simulink model "MSRE_final"  (R2017a)
settings: Solver=ode45  StartTime=0.0  StopTime=1500
values from neighbouring files (symbols this model uses):
  a_f = -11.034E-5    (= -0.00011034)    [Parameters_MSRE_cold_slug_U233.m]    (also in Parameters_MSRE_cold_slug_U235.m = -8.71e-05; Parameters_MSRE_pump_trip.m = -8.46e-05)
  a_g = -5.814E-5    (= -5.814e-05)    [Parameters_MSRE_cold_slug_U233.m]    (also in Parameters_MSRE_cold_slug_U235.m = -6.66e-05; Parameters_MSRE_pump_trip.m = -4.68e-05)
  beta = [0.00023,0.00079,0.00067,0.00073,0.00013,0.00009]    [Parameters_MSRE_cold_slug_U233.m]    (also in Parameters_MSRE_cold_slug_U235.m = [0.000223,0.001457,0.001307,0.002628,0.000766,0.00023]; Parameters_MSRE_pump_trip.m = [0.000215,0.00142,0.00127,0.00257,0.00075,0.00027])
  beta_t = sum(beta)    [Parameters_MSRE_cold_slug_U233.m]    (also in Parameters_MSRE_cold_slug_U235.m; Parameters_MSRE_pump_trip.m)
  hA_fg = 0.02*9/5    (= 0.036)    [Parameters_MSRE_cold_slug_U233.m]    (also in Parameters_MSRE_cold_slug_U235.m; Parameters_MSRE_pump_trip.m)
  hA_pn = ha_p/nn_s    (= 0.162)    [Parameters_MSRE_cold_slug_U233.m]    (also in Parameters_MSRE_cold_slug_U235.m; Parameters_MSRE_pump_trip.m)
  hA_rpn = h_roverall*A_rad/nn_rs    (= 0.0170417629704)    [Parameters_MSRE_cold_slug_U233.m]    (also in Parameters_MSRE_cold_slug_U235.m; Parameters_MSRE_pump_trip.m = 0.0166958844645)
  hA_rsn = h_roverall*A_rad/nn_rs    (= 0.0170417629704)    [Parameters_MSRE_cold_slug_U233.m]    (also in Parameters_MSRE_cold_slug_U235.m; Parameters_MSRE_pump_trip.m = 0.0166958844645)
  hA_sn = ha_s/nn_s    (= 0.0765)    [Parameters_MSRE_cold_slug_U233.m]    (also in Parameters_MSRE_cold_slug_U235.m; Parameters_MSRE_pump_trip.m)
  k_1 = 0.5    [Parameters_MSRE_cold_slug_U233.m]    (also in Parameters_MSRE_cold_slug_U235.m; Parameters_MSRE_pump_trip.m)
  k_2 = 0.5    [Parameters_MSRE_cold_slug_U233.m]    (also in Parameters_MSRE_cold_slug_U235.m; Parameters_MSRE_pump_trip.m)
  k_f1 = k_f/nn_f    (= 0.465)    [Parameters_MSRE_cold_slug_U233.m]    (also in Parameters_MSRE_cold_slug_U235.m; Parameters_MSRE_pump_trip.m)
  k_f2 = k_f/nn_f    (= 0.465)    [Parameters_MSRE_cold_slug_U233.m]    (also in Parameters_MSRE_cold_slug_U235.m; Parameters_MSRE_pump_trip.m)
  k_g = 0.07    [Parameters_MSRE_cold_slug_U233.m]    (also in Parameters_MSRE_cold_slug_U235.m; Parameters_MSRE_pump_trip.m)
  Lam = 4.0E-04    (= 0.0004)    [Parameters_MSRE_cold_slug_U233.m]    (also in Parameters_MSRE_cold_slug_U235.m = 0.00024; Parameters_MSRE_pump_trip.m = 0.00024)
  lam = [1.260E-02, 3.370E-02, 1.390E-01, 3.250E-01, 1.130E+00, 2.500E+00]    [Parameters_MSRE_cold_slug_U233.m]    (also in Parameters_MSRE_cold_slug_U235.m = [1.240E-02, 3.05E-02, 1.11E-01, 3.01E-01, 1.140E+00, 3.014E+; Parameters_MSRE_pump_trip.m)
  mcp_f1 = mn_f*scp_f    (= 1.52295504008)    [Parameters_MSRE_cold_slug_U233.m]    (also in Parameters_MSRE_cold_slug_U235.m; Parameters_MSRE_pump_trip.m = 1.32669270969)
  mcp_f2 = mn_f*scp_f    (= 1.52295504008)    [Parameters_MSRE_cold_slug_U233.m]    (also in Parameters_MSRE_cold_slug_U235.m; Parameters_MSRE_pump_trip.m = 1.32669270969)
  mcp_g1 = m_g*scp_g    (= 6.48)    [Parameters_MSRE_cold_slug_U233.m]    (also in Parameters_MSRE_cold_slug_U235.m; Parameters_MSRE_pump_trip.m)
  mcp_pn = mn_p*cp_p    (= 0.171274079686)    [Parameters_MSRE_cold_slug_U233.m]    (also in Parameters_MSRE_cold_slug_U235.m; Parameters_MSRE_pump_trip.m = 0.168097428848)
  mcp_rpn = mn_rp*cp_rp    (= 0.870039765806)    [Parameters_MSRE_cold_slug_U233.m]    (also in Parameters_MSRE_cold_slug_U235.m; Parameters_MSRE_pump_trip.m = 0.937931908109)
  mcp_rsn = mn_rs*scp_rs    (= 0.00358005261349)    [Parameters_MSRE_cold_slug_U233.m]    (also in Parameters_MSRE_cold_slug_U235.m; Parameters_MSRE_pump_trip.m)
  mcp_sn = mn_s*scp_s    (= 0.055247682268)    [Parameters_MSRE_cold_slug_U233.m]    (also in Parameters_MSRE_cold_slug_U235.m; Parameters_MSRE_pump_trip.m = 0.0595588455663)
  mcp_tn = m_tn*scp_t    (= 0.058453833323)    [Parameters_MSRE_cold_slug_U233.m]    (also in Parameters_MSRE_cold_slug_U235.m; Parameters_MSRE_pump_trip.m)
  mn_f = m_f/nn_f    (= 774.44955)    [Parameters_MSRE_cold_slug_U233.m]    (also in Parameters_MSRE_cold_slug_U235.m; Parameters_MSRE_pump_trip.m = 687.40554906)
  mn_p = m_p/nn_p    (= 87.0958961026)    [Parameters_MSRE_cold_slug_U233.m]    (also in Parameters_MSRE_cold_slug_U235.m; Parameters_MSRE_pump_trip.m = 87.0971133928)
  mn_rp = m_rp/nn_rp    (= 392.440128916)    [Parameters_MSRE_cold_slug_U233.m]    (also in Parameters_MSRE_cold_slug_U235.m; Parameters_MSRE_pump_trip.m)
  mn_rs = m_rs/nn_rs    (= 3.549878645)    [Parameters_MSRE_cold_slug_U233.m]    (also in Parameters_MSRE_cold_slug_U235.m; Parameters_MSRE_pump_trip.m)
  mn_s = m_s/nn_s    (= 24.9200190654)    [Parameters_MSRE_cold_slug_U233.m]    (also in Parameters_MSRE_cold_slug_U235.m; Parameters_MSRE_pump_trip.m)
  n_frac0 = 1    [Parameters_MSRE_cold_slug_U233.m]    (also in Parameters_MSRE_cold_slug_U235.m; Parameters_MSRE_pump_trip.m)
  P = 8    [Parameters_MSRE_cold_slug_U233.m]    (also in Parameters_MSRE_cold_slug_U235.m; Parameters_MSRE_pump_trip.m)
  T0_f1 = Tf_in + (T0_f2-Tf_in)/2    (= 643.33)    [Parameters_MSRE_cold_slug_U233.m]    (also in Parameters_MSRE_cold_slug_U235.m; Parameters_MSRE_pump_trip.m = 648.9)
  T0_f2 = 6.5444E+02    (= 654.44)    [Parameters_MSRE_cold_slug_U233.m]    (also in Parameters_MSRE_cold_slug_U235.m; Parameters_MSRE_pump_trip.m = 662.8)
  T0_g1 = T0_f1+(k_g*P/hA_fg)    (= 658.885555556)    [Parameters_MSRE_cold_slug_U233.m]    (also in Parameters_MSRE_cold_slug_U235.m; Parameters_MSRE_pump_trip.m = 664.455555556)
  T0_p1 = Tp_in - (Tp_in-T0_p4)/4    (= 648.885)    [Parameters_MSRE_cold_slug_U233.m]    (also in Parameters_MSRE_cold_slug_U235.m; Parameters_MSRE_pump_trip.m = 655.85)
  T0_p2 = Tp_in - 2*(Tp_in-T0_p4)/4    (= 643.33)    [Parameters_MSRE_cold_slug_U233.m]    (also in Parameters_MSRE_cold_slug_U235.m; Parameters_MSRE_pump_trip.m = 648.9)
  T0_p3 = Tp_in - 3*(Tp_in-T0_p4)/4    (= 637.775)    [Parameters_MSRE_cold_slug_U233.m]    (also in Parameters_MSRE_cold_slug_U235.m; Parameters_MSRE_pump_trip.m = 641.95)
  T0_p4 = Tf_in    (= 632.22)    [Parameters_MSRE_cold_slug_U233.m]    (also in Parameters_MSRE_cold_slug_U235.m; Parameters_MSRE_pump_trip.m = 635)
  T0_rp = Ts_in    (= 546.11)    [Parameters_MSRE_cold_slug_U233.m]    (also in Parameters_MSRE_cold_slug_U235.m; Parameters_MSRE_pump_trip.m = 551.7)
  T0_rs = 148.9    [Parameters_MSRE_cold_slug_U233.m]    (also in Parameters_MSRE_cold_slug_U235.m; Parameters_MSRE_pump_trip.m)
  T0_s1 = Ts_in + (T0_s4-Ts_in)/nn_s    (= 554.4425)    [Parameters_MSRE_cold_slug_U233.m]    (also in Parameters_MSRE_cold_slug_U235.m; Parameters_MSRE_pump_trip.m = 562.1)
  T0_s2 = Ts_in + 2*(T0_s4-Ts_in)/nn_s    (= 562.775)    [Parameters_MSRE_cold_slug_U233.m]    (also in Parameters_MSRE_cold_slug_U235.m; Parameters_MSRE_pump_trip.m = 572.5)
  T0_s3 = Ts_in + 3*(T0_s4-Ts_in)/nn_s    (= 571.1075)    [Parameters_MSRE_cold_slug_U233.m]    (also in Parameters_MSRE_cold_slug_U235.m; Parameters_MSRE_pump_trip.m = 582.9)
  T0_s4 = 5.7944E+02    (= 579.44)    [Parameters_MSRE_cold_slug_U233.m]    (also in Parameters_MSRE_cold_slug_U235.m; Parameters_MSRE_pump_trip.m = 593.3)
  T0_t1 = (T0_p1*hA_pn+T0_s3*hA_sn)/(hA_pn+hA_sn)    (= 623.9375)    [Parameters_MSRE_cold_slug_U233.m]    (also in Parameters_MSRE_cold_slug_U235.m; Parameters_MSRE_pump_trip.m = 632.450943396)
  T0_t2 = (T0_p3*hA_pn+T0_s1*hA_sn)/(hA_pn+hA_sn)    (= 611.045707547)    [Parameters_MSRE_cold_slug_U233.m]    (also in Parameters_MSRE_cold_slug_U235.m; Parameters_MSRE_pump_trip.m = 616.337735849)
  tau_c = 8.46    [Parameters_MSRE_cold_slug_U233.m]    (also in Parameters_MSRE_cold_slug_U235.m; Parameters_MSRE_pump_trip.m)
  tau_c_hx = 3.77    [Parameters_MSRE_cold_slug_U233.m]    (also in Parameters_MSRE_cold_slug_U235.m; Parameters_MSRE_pump_trip.m)
  tau_hx_c = 8.67    [Parameters_MSRE_cold_slug_U233.m]    (also in Parameters_MSRE_cold_slug_U235.m; Parameters_MSRE_pump_trip.m)
  tau_hx_r = 4.71    [Parameters_MSRE_cold_slug_U233.m]    (also in Parameters_MSRE_cold_slug_U235.m; Parameters_MSRE_pump_trip.m)
  tau_l = 16.73    [Parameters_MSRE_cold_slug_U233.m]    (also in Parameters_MSRE_cold_slug_U235.m; Parameters_MSRE_pump_trip.m)
  tau_r_hx = 8.24    [Parameters_MSRE_cold_slug_U233.m]    (also in Parameters_MSRE_cold_slug_U235.m; Parameters_MSRE_pump_trip.m)
  Trs_in = 37.78    [Parameters_MSRE_cold_slug_U233.m]    (also in Parameters_MSRE_cold_slug_U235.m; Parameters_MSRE_pump_trip.m)
  W_f = 1.83085e+02    (= 183.085)    [Parameters_MSRE_cold_slug_U233.m]    (also in Parameters_MSRE_cold_slug_U235.m; Parameters_MSRE_pump_trip.m = 162.507222)
  W_p = W_f    (= 183.085)    [Parameters_MSRE_cold_slug_U233.m]    (also in Parameters_MSRE_cold_slug_U235.m; Parameters_MSRE_pump_trip.m = 162.507222)
  W_rp = W_s    (= 108.27)    [Parameters_MSRE_cold_slug_U233.m]    (also in Parameters_MSRE_cold_slug_U235.m; Parameters_MSRE_pump_trip.m = 100.579336981)
  W_rs = vdot_rs*rho_rs    (= 106.0649193)    [Parameters_MSRE_cold_slug_U233.m]    (also in Parameters_MSRE_cold_slug_U235.m; Parameters_MSRE_pump_trip.m)
  W_s = 1.0827e+02    (= 108.27)    [Parameters_MSRE_cold_slug_U233.m]    (also in Parameters_MSRE_cold_slug_U235.m; Parameters_MSRE_pump_trip.m = 100.579336981)
undefined symbols (not defined in the file or in its folder): C0
libraries: simulink x1
settings Model: Creator=mlish  LastModifiedBy=awheel13

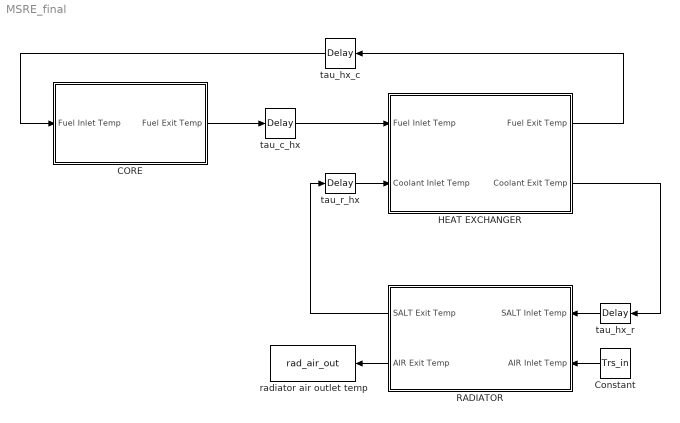
== system MSRE_final ==
  " HEAT EXCHANGER" : Subsystem
  CORE : Subsystem
  Constant : Constant  Value=Trs_in
  RADIATOR : Subsystem
  radiator air outlet temp : ToWorkspace  VariableName=rad_air_out  SampleTime=-1
  tau_c_hx : TransportDelay  DelayTime=tau_c_hx  InitialOutput=T0_f2  BufferSize=4096
  tau_hx_c : TransportDelay  DelayTime=tau_hx_c  InitialOutput=T0_p4  BufferSize=4096
  tau_hx_r : TransportDelay  DelayTime=tau_hx_r  InitialOutput=T0_s4  BufferSize=4096
  tau_r_hx : TransportDelay  DelayTime=tau_r_hx  InitialOutput=T0_rp  BufferSize=4096
  wires:
  tau_hx_r/1 -> RADIATOR/1(SALT Inlet Temp)
  " HEAT EXCHANGER"/1(Fuel Exit Temp) -> tau_hx_c/1
  RADIATOR/1(SALT Exit Temp) -> tau_r_hx/1
  tau_c_hx/1 -> " HEAT EXCHANGER"/1(Fuel Inlet Temp)
  Constant/1 -> RADIATOR/2(AIR Inlet Temp)
  RADIATOR/2(AIR Exit Temp) -> radiator air outlet temp/1
  tau_r_hx/1 -> " HEAT EXCHANGER"/2(Coolant Inlet Temp)
  " HEAT EXCHANGER"/2(Coolant Exit Temp) -> tau_hx_r/1
  tau_hx_c/1 -> CORE/1(Fuel Inlet Temp)
  CORE/1(Fuel Exit Temp) -> tau_c_hx/1

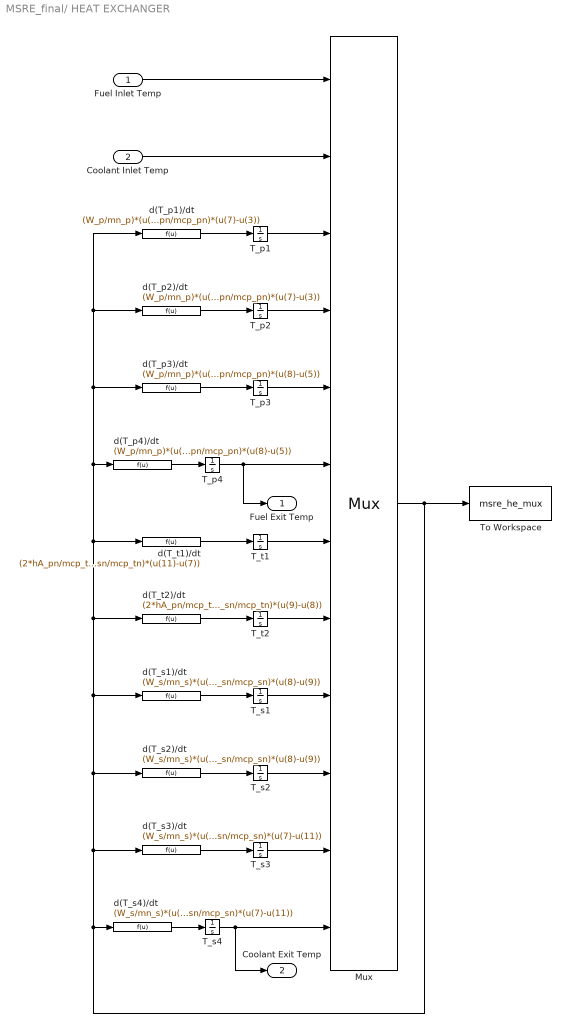
== system MSRE_final/ HEAT EXCHANGER ==
  Fuel Inlet Temp : Inport
  Coolant Inlet Temp : Inport  Port=2
  Mux : Mux  Inputs=12
      settings: DisplayOption=signals
  T_p1 : Integrator  InitialCondition=T0_p1
  T_p2 : Integrator  InitialCondition=T0_p2
  "T_p3 " : Integrator  InitialCondition=T0_p3
  T_p4 : Integrator  InitialCondition=T0_p4
  T_s1 : Integrator  InitialCondition=T0_s1
  T_s2 : Integrator  InitialCondition=T0_s2
  T_s3 : Integrator  InitialCondition=T0_s3
  T_s4 : Integrator  InitialCondition=T0_s4
  T_t1 : Integrator  InitialCondition=T0_t1
  T_t2 : Integrator  InitialCondition=T0_t2
  To Workspace : ToWorkspace  VariableName=msre_he_mux  SampleTime=-1
  d(T_p1)/dt : Fcn  Expr=(W_p/mn_p)*(u(1)-u(3)) + (hA_pn/mcp_pn)*(u(7)-u(3))
  d(T_p2)/dt : Fcn  Expr=(W_p/mn_p)*(u(3)-u(4)) + (hA_pn/mcp_pn)*(u(7)-u(3))
  d(T_p3)/dt : Fcn  Expr=(W_p/mn_p)*(u(4)-u(5)) + (hA_pn/mcp_pn)*(u(8)-u(5))
  d(T_p4)/dt : Fcn  Expr=(W_p/mn_p)*(u(5)-u(6)) + (hA_pn/mcp_pn)*(u(8)-u(5))
  d(T_s1)/dt : Fcn  Expr=(W_s/mn_s)*(u(2)-u(9)) + (hA_sn/mcp_sn)*(u(8)-u(9))
  d(T_s2)/dt : Fcn  Expr=(W_s/mn_s)*(u(9)-u(10)) + (hA_sn/mcp_sn)*(u(8)-u(9))
  d(T_s3)/dt : Fcn  Expr=(W_s/mn_s)*(u(10)-u(11)) + (hA_sn/mcp_sn)*(u(7)-u(11))
  d(T_s4)/dt : Fcn  Expr=(W_s/mn_s)*(u(11)-u(12)) + (hA_sn/mcp_sn)*(u(7)-u(11))
  d(T_t1)/dt : Fcn  Expr=(2*hA_pn/mcp_tn)*(u(3)-u(7)) + (2*hA_sn/mcp_tn)*(u(11)-u(7))
  d(T_t2)/dt : Fcn  Expr=(2*hA_pn/mcp_tn)*(u(5)-u(8)) + (2*hA_sn/mcp_tn)*(u(9)-u(8))
  Fuel Exit Temp : Outport
  Coolant Exit Temp : Outport  Port=2
  wires:
  Fuel Inlet Temp/1 -> Mux/1
  Coolant Inlet Temp/1 -> Mux/2
  d(T_p1)/dt/1 -> T_p1/1
  d(T_p2)/dt/1 -> T_p2/1
  d(T_p3)/dt/1 -> "T_p3 "/1
  d(T_p4)/dt/1 -> T_p4/1
  d(T_t1)/dt/1 -> T_t1/1
  d(T_t2)/dt/1 -> T_t2/1
  d(T_s1)/dt/1 -> T_s1/1
  d(T_s2)/dt/1 -> T_s2/1
  T_p2/1 -> Mux/4
  T_p1/1 -> Mux/3
  d(T_s3)/dt/1 -> T_s3/1
  d(T_s4)/dt/1 -> T_s4/1
  Mux/1 -> d(T_s4)/dt/1, d(T_s3)/dt/1, d(T_s2)/dt/1, d(T_s1)/dt/1, d(T_t2)/dt/1, d(T_t1)/dt/1, d(T_p4)/dt/1, d(T_p3)/dt/1, d(T_p2)/dt/1, d(T_p1)/dt/1, To Workspace/1
  "T_p3 "/1 -> Mux/5
  T_p4/1 -> Fuel Exit Temp/1, Mux/6
  T_t1/1 -> Mux/7
  T_s4/1 -> Coolant Exit Temp/1, Mux/12
  T_s3/1 -> Mux/11
  T_s2/1 -> Mux/10
  T_s1/1 -> Mux/9
  T_t2/1 -> Mux/8

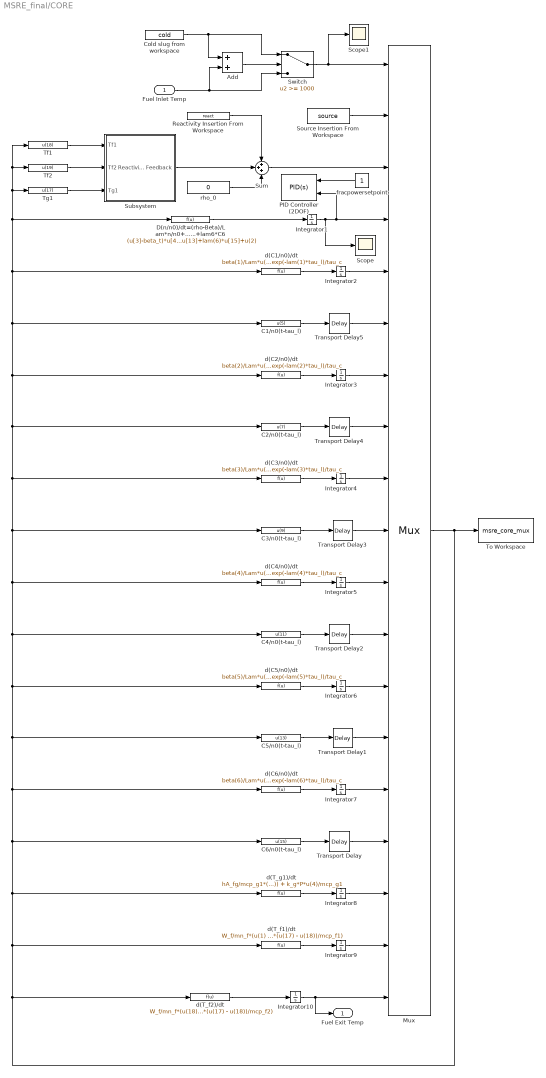
== system MSRE_final/CORE ==
  Fuel Inlet Temp : Inport
  Add : Sum
  C1/n0(t-tau_l) : Fcn  Expr=u(5)
  C2/n0(t-tau_l) : Fcn  Expr=u(7)
  C3/n0(t-tau_l) : Fcn  Expr=u(9)
  C4/n0(t-tau_l) : Fcn  Expr=u(11)
  C5/n0(t-tau_l) : Fcn  Expr=u(13)
  C6/n0(t-tau_l) : Fcn  Expr=u(15)
  Cold slug from workspace : FromWorkspace  VariableName=cold  SampleTime=1  Interpolate=off  OutputAfterFinalValue=Holding final value
  D(n/n0)/dt=(rho-Beta)/Lam*n/n0+lam1*C1+...+lam6*C6 : Fcn  Expr=(u[3]-beta_t)*u[4]/Lam+lam(1)*u[5]+lam(2)*u[7]+lam(3)*u[9]+lam(4)*u[11]+lam(5)*u[13]+lam(6)*u[15]+u(2)
  Integrator1 : Integrator  InitialCondition=n_frac0
  Integrator10 : Integrator  InitialCondition=T0_f2
  Integrator2 : Integrator  InitialCondition=C0(1)
  Integrator3 : Integrator  InitialCondition=C0(2)
  Integrator4 : Integrator  InitialCondition=C0(3)
  Integrator5 : Integrator  InitialCondition=C0(4)
  Integrator6 : Integrator  InitialCondition=C0(5)
  Integrator7 : Integrator  InitialCondition=C0(6)
  Integrator8 : Integrator  InitialCondition=T0_g1
  Integrator9 : Integrator  InitialCondition=T0_f1
  Mux : Mux  Inputs=19
      settings: DisplayOption=signals
  PID Controller (2DOF) : simulink/Continuous/PID Controller (2DOF)  Controller=PID  TimeDomain=Continuous-time  SampleTime=-1  IntegratorMethod=Forward Euler  FilterMethod=Forward Euler  Form=Parallel  UseFilter=on  ControllerParametersSource=internal  P=0.00795461875019384  I=0.16107974098195  D=-5.4273429935444e-05  N=35.3820871609057  b=0.816735959251165  c=1.20544692397769  InitialConditionSource=internal  InitialConditionForIntegrator=0  InitialConditionForFilter=0  ExternalReset=none  LimitOutput=off  UpperSaturationLimit=inf  LowerSaturationLimit=-inf  LinearizeAsGain=on  AntiWindupMode=none  Kb=1  TrackingMode=off  Kt=1  PParamMin=[]  PParamMax=[]  IParamMin=[]  IParamMax=[]  DParamMin=[]  DParamMax=[]  NParamMin=[]  NParamMax=[]  bParamMin=[]  bParamMax=[]  cParamMin=[]  cParamMax=[]  KbParamMin=[]  KbParamMax=[]  KtParamMin=[]  KtParamMax=[]  POutMin=[]  POutMax=[]  IOutMin=[]  IOutMax=[]  DOutMin=[]  DOutMax=[]  NOutMin=[]  NOutMax=[]  bOutMin=[]  bOutMax=[]  cOutMin=[]  cOutMax=[]  KbOutMin=[]  KbOutMax=[]  KtOutMin=[]  KtOutMax=[]  IntegratorOutMin=[]  IntegratorOutMax=[]  FilterOutMin=[]  FilterOutMax=[]  SumOutMin=[]  SumOutMax=[]  Sum1OutMin=[]  Sum1OutMax=[]  Sum2OutMin=[]  Sum2OutMax=[]  Sum3OutMin=[]  Sum3OutMax=[]  SumI1OutMin=[]  SumI1OutMax=[]  SumI2OutMin=[]  SumI2OutMax=[]  SumI3OutMin=[]  SumI3OutMax=[]  SumDOutMin=[]  SumDOutMax=[]  SaturationOutMin=[]  SaturationOutMax=[]  IntegratorContinuousStateAttributes=''  IntegratorStateMustResolveToSignalObject=off  IntegratorRTWStateStorageClass=Auto  FilterContinuousStateAttributes=''  FilterStateMustResolveToSignalObject=off  FilterRTWStateStorageClass=Auto  DifferentiatorICPrevScaledInput=0  DifferentiatorOutMin=[]  DifferentiatorOutMax=[]  InitialConditionSetting=State (most efficient)
  Reactivity Insertion From Workspace : FromWorkspace  VariableName=react  SampleTime=1  Interpolate=off  OutputAfterFinalValue=Holding final value
  Scope : Scope
  Scope1 : Scope
  Source Insertion From Workspace : FromWorkspace  VariableName=source  SampleTime=1  Interpolate=off  OutputAfterFinalValue=Holding final value
  Subsystem : Subsystem
  Sum : Sum  Inputs=+++
  Switch : Switch  Threshold=1000
  Tf1 : Fcn  Expr=u(18)
  Tf2 : Fcn  Expr=u(19)
  Tg1 : Fcn  Expr=u(17)
  To Workspace : ToWorkspace  VariableName=msre_core_mux  SampleTime=-1
  Transport Delay : TransportDelay  DelayTime=tau_l  InitialOutput=C0(6)  BufferSize=4096
  Transport Delay1 : TransportDelay  DelayTime=tau_l  InitialOutput=C0(5)  BufferSize=4096
  Transport Delay2 : TransportDelay  DelayTime=tau_l  InitialOutput=C0(4)  BufferSize=4096
  Transport Delay3 : TransportDelay  DelayTime=tau_l  InitialOutput=C0(3)  BufferSize=4096
  Transport Delay4 : TransportDelay  DelayTime=tau_l  InitialOutput=C0(2)  BufferSize=4096
  Transport Delay5 : TransportDelay  DelayTime=tau_l  InitialOutput=C0(1)  BufferSize=4096
  d(C1/n0)/dt : Fcn  Expr=beta(1)/Lam*u(4)-lam(1)*u(5)-u(5)/tau_c+u(6)*exp(-lam(1)*tau_l)/tau_c
  d(C2/n0)/dt : Fcn  Expr=beta(2)/Lam*u(4)-lam(2)*u(7)-u(7)/tau_c+u(8)*exp(-lam(2)*tau_l)/tau_c
  d(C3/n0)/dt : Fcn  Expr=beta(3)/Lam*u(4)-lam(3)*u(9)-u(9)/tau_c+u(10)*exp(-lam(3)*tau_l)/tau_c
  d(C4/n0)/dt : Fcn  Expr=beta(4)/Lam*u(4)-lam(4)*u(11)-u(11)/tau_c+u(12)*exp(-lam(4)*tau_l)/tau_c
  d(C5/n0)/dt : Fcn  Expr=beta(5)/Lam*u(4)-lam(5)*u(13)-u(13)/tau_c+u(14)*exp(-lam(5)*tau_l)/tau_c
  d(C6/n0)/dt : Fcn  Expr=beta(6)/Lam*u(4)-lam(6)*u(15)-u(15)/tau_c+u(16)*exp(-lam(6)*tau_l)/tau_c
  d(T_f1)/dt : Fcn  Expr=W_f/mn_f*(u(1) - u(18)) + (k_f1*P*u(4)/mcp_f1) + (hA_fg*k_1*(u(17) - u(18))/mcp_f1)
  d(T_f2)/dt : Fcn  Expr=W_f/mn_f*(u(18) - u(19)) + (k_f2*P*u(4)/mcp_f2) + (hA_fg*k_2*(u(17) - u(18))/mcp_f2)
  d(T_g1)/dt : Fcn  Expr=hA_fg/mcp_g1*(u(18) - u(17)) + k_g*P*u(4)/mcp_g1
  fracpowersetpoint : Constant
  rho_0 : Constant  Value=0
  Fuel Exit Temp : Outport
  wires:
  Transport Delay3/1 -> Mux/10
  C3/n0(t-tau_l)/1 -> Transport Delay3/1
  Transport Delay4/1 -> Mux/8
  C4/n0(t-tau_l)/1 -> Transport Delay2/1
  Integrator7/1 -> Mux/15
  Transport Delay2/1 -> Mux/12
  C5/n0(t-tau_l)/1 -> Transport Delay1/1
  Transport Delay/1 -> Mux/16
  Transport Delay1/1 -> Mux/14
  C6/n0(t-tau_l)/1 -> Transport Delay/1
  D(n/n0)/dt=(rho-Beta)/Lam*n/n0+lam1*C1+...+lam6*C6/1 -> Integrator1/1
  fracpowersetpoint/1 -> PID Controller (2DOF)/1
  Integrator10/1 -> Fuel Exit Temp/1, Mux/19
  d(C5/n0)/dt/1 -> Integrator6/1
  d(C3/n0)/dt/1 -> Integrator4/1
  d(C2/n0)/dt/1 -> Integrator3/1
  d(C4/n0)/dt/1 -> Integrator5/1
  d(C1/n0)/dt/1 -> Integrator2/1
  C2/n0(t-tau_l)/1 -> Transport Delay4/1
  Source Insertion From Workspace/1 -> Mux/2
  C1/n0(t-tau_l)/1 -> Transport Delay5/1
  Mux/1 -> d(T_f2)/dt/1, d(T_f1)/dt/1, d(T_g1)/dt/1, C6/n0(t-tau_l)/1, d(C6/n0)/dt/1, C5/n0(t-tau_l)/1, d(C5/n0)/dt/1, C4/n0(t-tau_l)/1, d(C4/n0)/dt/1, C3/n0(t-tau_l)/1, d(C3/n0)/dt/1, d(C2/n0)/dt/1, C1/n0(t-tau_l)/1, D(n/n0)/dt=(rho-Beta)/Lam*n/n0+lam1*C1+...+lam6*C6/1, Tf1/1, Tf2/1, Tg1/1, d(C1/n0)/dt/1, C2/n0(t-tau_l)/1, To Workspace/1
  Transport Delay5/1 -> Mux/6
  d(C6/n0)/dt/1 -> Integrator7/1
  Integrator5/1 -> Mux/11
  Integrator3/1 -> Mux/7
  Integrator2/1 -> Mux/5
  Integrator4/1 -> Mux/9
  Integrator1/1 -> Scope/1, Mux/4, PID Controller (2DOF)/2
  Integrator6/1 -> Mux/13
  d(T_f2)/dt/1 -> Integrator10/1
  d(T_f1)/dt/1 -> Integrator9/1
  Integrator9/1 -> Mux/18
  d(T_g1)/dt/1 -> Integrator8/1
  Integrator8/1 -> Mux/17
  Tf1/1 -> Subsystem/1(Tf1)
  Tg1/1 -> Subsystem/3(Tg1)
  Tf2/1 -> Subsystem/2(Tf2)
  rho_0/1 -> Sum/3
  Sum/1 -> Mux/3
  Subsystem/1(Reactivity Feedback) -> Sum/2
  Reactivity Insertion From Workspace/1 -> Sum/1
  Switch/1 -> Scope1/1, Mux/1
  Add/1 -> Switch/2
  Fuel Inlet Temp/1 -> Add/2, Switch/3
  Cold slug from workspace/1 -> Add/1, Switch/1

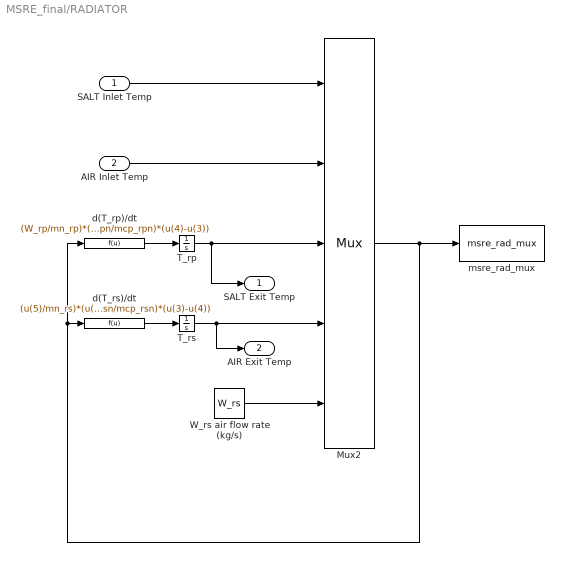
== system MSRE_final/RADIATOR ==
  SALT Inlet Temp : Inport
  AIR Inlet Temp : Inport  Port=2
  Mux2 : Mux  Inputs=5
      settings: DisplayOption=signals
  T_rp : Integrator  InitialCondition=T0_rp
  T_rs : Integrator  InitialCondition=T0_rs
  W_rs air flow rate (kg/s) : Constant  Value=W_rs
  d(T_rp)/dt : Fcn  Expr=(W_rp/mn_rp)*(u(1)-u(3)) + (hA_rpn/mcp_rpn)*(u(4)-u(3))
  d(T_rs)/dt : Fcn  Expr=(u(5)/mn_rs)*(u(2)-u(4)) + (hA_rsn/mcp_rsn)*(u(3)-u(4))
  msre_rad_mux : ToWorkspace  VariableName=msre_rad_mux  SampleTime=-1
  SALT Exit Temp : Outport
  AIR Exit Temp : Outport  Port=2
  wires:
  SALT Inlet Temp/1 -> Mux2/1
  AIR Inlet Temp/1 -> Mux2/2
  d(T_rp)/dt/1 -> T_rp/1
  T_rp/1 -> Mux2/3, SALT Exit Temp/1
  d(T_rs)/dt/1 -> T_rs/1
  T_rs/1 -> Mux2/4, AIR Exit Temp/1
  Mux2/1 -> d(T_rs)/dt/1, d(T_rp)/dt/1, msre_rad_mux/1
  W_rs air flow rate (kg/s)/1 -> Mux2/5

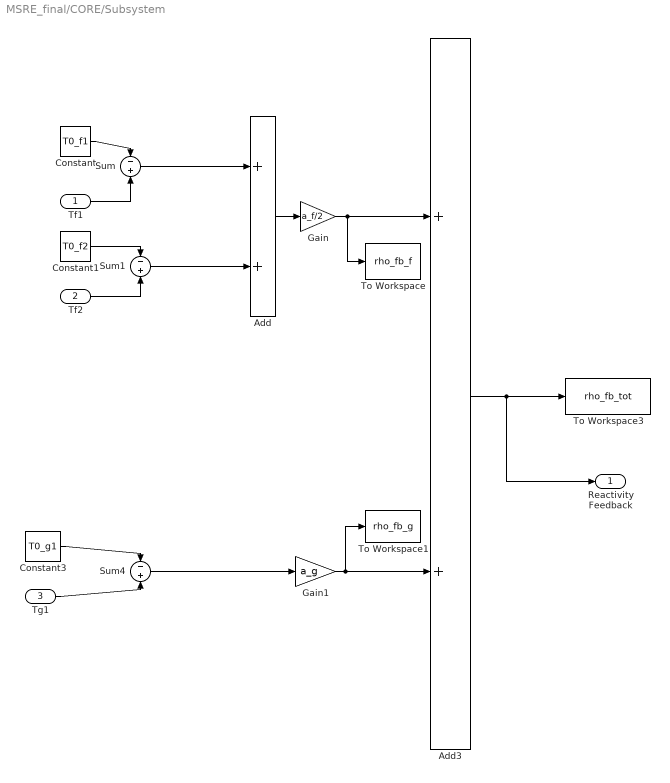
== system MSRE_final/CORE/Subsystem ==
  Tf1 : Inport
  Tf2 : Inport  Port=2
  Tg1 : Inport  Port=3
  Add : Sum
  Add3 : Sum
  Constant : Constant  Value=T0_f1
  Constant1 : Constant  Value=T0_f2
  Constant3 : Constant  Value=T0_g1
  Gain : Gain  Gain=a_f/2
  Gain1 : Gain  Gain=a_g
  Sum : Sum  Inputs=-|+
  Sum1 : Sum  Inputs=-|+
  Sum4 : Sum  Inputs=-|+
  To Workspace : ToWorkspace  VariableName=rho_fb_f  SampleTime=-1
  To Workspace1 : ToWorkspace  VariableName=rho_fb_g  SampleTime=-1
  To Workspace3 : ToWorkspace  VariableName=rho_fb_tot  SampleTime=-1
  Reactivity Feedback : Outport
  wires:
  Tf1/1 -> Sum/2
  Constant/1 -> Sum/1
  Tf2/1 -> Sum1/2
  Constant1/1 -> Sum1/1
  Tg1/1 -> Sum4/2
  Constant3/1 -> Sum4/1
  Sum/1 -> Add/1
  Sum1/1 -> Add/2
  Add/1 -> Gain/1
  Sum4/1 -> Gain1/1
  Gain1/1 -> To Workspace1/1, Add3/2
  Gain/1 -> Add3/1, To Workspace/1
  Add3/1 -> Reactivity Feedback/1, To Workspace3/1
